simulink model "base_model"  (R2022a)
settings: Solver=ode23t  StartTime=0.0  StopTime=2  RelTol=1e-3
model workspace (MAT data in the model file):
  Kp_MPPT = 1.14714733987
  Ts_Control = 0.0001
  Ts_MPPT = 0.0001
undefined symbols (not defined in the file): Ion, Lithium, load_switch
libraries: spsSeriesRLCBranchLib x13, simulink x6, spsCurrentMeasurementLib x5, spsVoltageMeasurementLib x4, slpidlib x3, spsIGBTDiodeLib x2, spsDiodeLib x2, spsMosfetLib x2, spsPWMGeneratorDCDCLib x2, spsPVArrayLib x2, spsBatteryLib x1, spsIdealSwitchLib x1
settings Model: Creator=drmeg  LastModifiedBy=drmeg
settings SolverCC: ZeroCrossAlgorithm=Adaptive
settings OptimizationCC: ZeroExternalMemoryAtStartup=off  ZeroInternalMemoryAtStartup=off
settings DebuggingCC: MaskedZcDiagnostic=none  IgnoredZcDiagnostic=none  UnconnectedInputMsg=warning  UnconnectedOutputMsg=warning  UnconnectedLineMsg=warning
settings RTWCC: TargetLang=C++  DLArmComputeVersion=19.05
settings GRTTargetCC: TargetLangStandard=C++11 (ISO)  CodeInterfacePackaging=C++ class

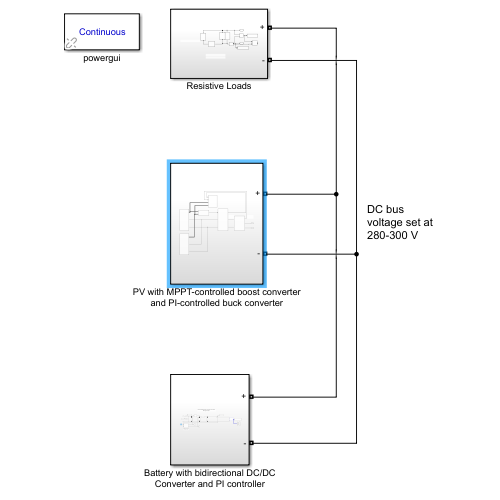
[thumbnail: Simulink's stored preview of the top-level diagram]
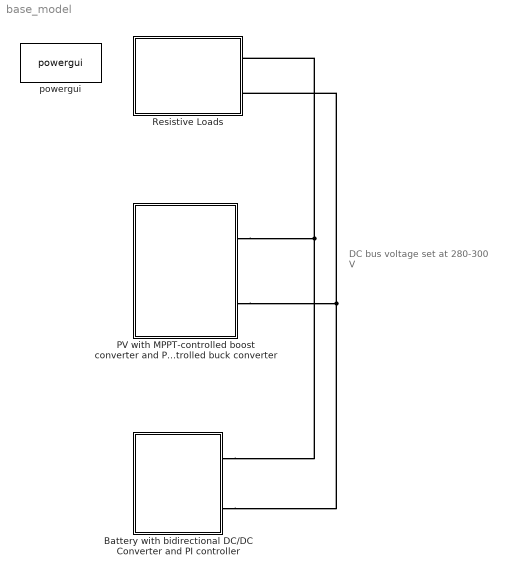
== system base_model ==
  note: DC bus voltage set at
      | 280-300 V
  Battery with bidirectional DC/DC Converter and PI controller : Subsystem
  PV with MPPT-controlled boost converter and PI-controlled buck converter : Subsystem
  Resistive Loads : Subsystem
  powergui : spspowerguiLib/powergui  Priority=1  SimulationMode=Continuous  SampleTime=1e-6  frequency=60  Iterations=50  frequencyindice=0  Pbase=100e6  ErrMax=1e-4  UnitsV=kV  UnitsW=MW  buscounter=0  FunctionMessages=off  echomessages=off  EnableUseOfTLC=off  CurrentSourceSwitches=off  DisableSnubberDevices=off  DisableRonSwitches=off  DisableVfSwitches=off  DisplayEquations=off  AutomaticDiscreteSolvers=off  SolverType=Tustin/Backward Euler (TBE)  Interpol=off  ExternalGateDelay=off  methode=off  Ts=100  x0status=blocks  SPID=on  SwTol=0  HookPort=off  NonlinearTolerance=1e-4  nMaxIteration=100  ContinueOnMaxIteration=off  RestoreLinks=warning  ResistiveCurrentMeasurement=off  Frange=[0:2:500]  Ylog=off  Xlog=on  ShowGrid=off  save=off  variable=ZData  structure=0  ZoomFFT=off  StartTime=0.0  cycles=1  DisplayStyle=1  fundamental=60  FreqAxis=off  MaxFrequency=1000  frequencyindicesteady=1  RmsSteady=1  display=off
  connections:
  Battery with bidirectional DC/DC Converter and PI controller/LConn2 -- Resistive Loads/RConn2 -- PV with MPPT-controlled boost converter and PI-controlled buck converter/RConn2
  Battery with bidirectional DC/DC Converter and PI controller/LConn1 -- Resistive Loads/RConn1 -- PV with MPPT-controlled boost converter and PI-controlled buck converter/RConn1

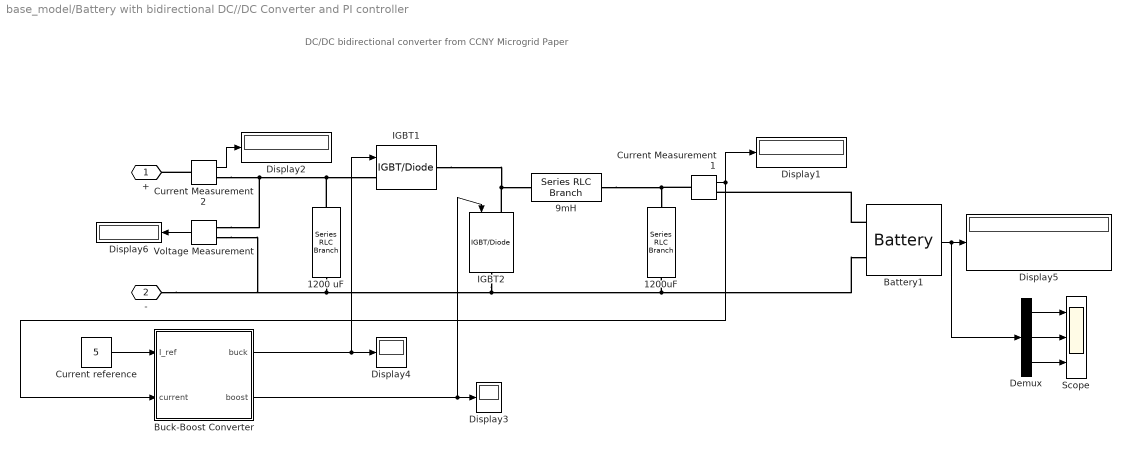
== system base_model/Battery with bidirectional DC//DC Converter and PI controller ==
  note: DC/DC bidirectional converter from CCNY Microgrid Paper
  1200 uF : spsSeriesRLCBranchLib/Series RLC Branch  LConnTagsString=__new0  RConnTagsString=__new0  BranchType=RC  Resistance=0.1  Inductance=3e-3  SetiL0=off  InitialCurrent=0  Capacitance=1200e-6  Setx0=off  InitialVoltage=0  Measurements=None
  1200uF : spsSeriesRLCBranchLib/Series RLC Branch  LConnTagsString=__new0  RConnTagsString=__new0  BranchType=C  Resistance=1  Inductance=3e-3  SetiL0=off  InitialCurrent=0  Capacitance=1200e-6  Setx0=off  InitialVoltage=0  Measurements=None
  9mH : spsSeriesRLCBranchLib/Series RLC Branch  LConnTagsString=__new0  RConnTagsString=__new0  BranchType=L  Resistance=1  Inductance=9e-3  SetiL0=off  InitialCurrent=0  Capacitance=1e-6  Setx0=off  InitialVoltage=0  Measurements=None
  Battery1 : spsBatteryLib/Battery  BatType=Lithium-Ion  ShowTempParam=off  ThermalPreset=no  ShowAgeParam=off  NomV=150  NomQ=80  SOC=100  Batt_Tr=3  PresetModel=on  MaxQ=80  MinV=112.5  FullV=174.5981  Dis_rate=34.7826  R=0.01875  Normal_OP=72.3478  expZone="[162.0579      3.930435]"  current=[1.5 3]  Units=Ampere-hour  Tci=20  NomT=25  T2=0  MaxQ2=2.208  FullV2=3.45  Normal_OP2=2.8  expZone2="[3.22        0.23]"  Rca=0.6  ti=1000  Dp=0  Neq0=0  Tsim=1e6  Ta1=25  Qeol=5.4*0.9  Reol=0.013333*1.2  Char_age=[2.3478, 3]  Dis_age=[2.3478, 10]  N1=1500  N2=10500  N3=1000  N4=1400  Ta2=45  N5=950
  Buck-Boost Converter : Subsystem
  Current Measurement1 : spsCurrentMeasurementLib/Current Measurement  PhasorSimulation=off  OutputType=Complex  PSBequivalent=0
  Current Measurement2 : spsCurrentMeasurementLib/Current Measurement  PhasorSimulation=off  OutputType=Complex  PSBequivalent=0
  Current reference : Constant  Value=5
  Demux : Demux  Outputs=3
  Display{1..6} (6 alike) : Display
      Display5 settings: Format=decimal (Stored Integer)
  IGBT1 : spsIGBTDiodeLib/IGBT//Diode  Ron=1e-3  Rs=1e5  Cs=inf  Measurements=off
  IGBT2 : spsIGBTDiodeLib/IGBT//Diode  Ron=1e-3  Rs=1e5  Cs=inf  Measurements=off
  Scope : Scope  NumInputPorts=3
  Voltage Measurement : spsVoltageMeasurementLib/Voltage Measurement  PhasorSimulation=off  OutputType=Complex  PSBequivalent=0
  + : PMIOPort  Side=Left
  - : PMIOPort  Port=2  Side=Left
  wires:
  Buck-Boost Converter/2(boost) -> Display3/1, IGBT2/1
  Current Measurement1/1 -> Display1/1, Buck-Boost Converter/2(current)
  Buck-Boost Converter/1(buck) -> Display4/1, IGBT1/1
  Current reference/1 -> Buck-Boost Converter/1(I_ref)
  Current Measurement2/1 -> Display2/1
  Battery1/1 -> Demux/1, Display5/1
  Voltage Measurement/1 -> Display6/1
  Demux/3 -> Scope/3
  Demux/2 -> Scope/2
  Demux/1 -> Scope/1
  connections:
  Current Measurement1/LConn1 -- 1200uF/LConn1 -- 9mH/RConn1
  1200uF/RConn1 -- Battery1/LConn2 -- IGBT2/RConn1 -- -/RConn1 -- Voltage Measurement/LConn2 -- 1200 uF/RConn1
  IGBT1/RConn1 -- 9mH/LConn1 -- IGBT2/LConn1
  Current Measurement2/RConn1 -- 1200 uF/LConn1 -- IGBT1/LConn1 -- Voltage Measurement/LConn1
  Battery1/LConn1 -- Current Measurement1/RConn1
  Current Measurement2/LConn1 -- +/RConn1

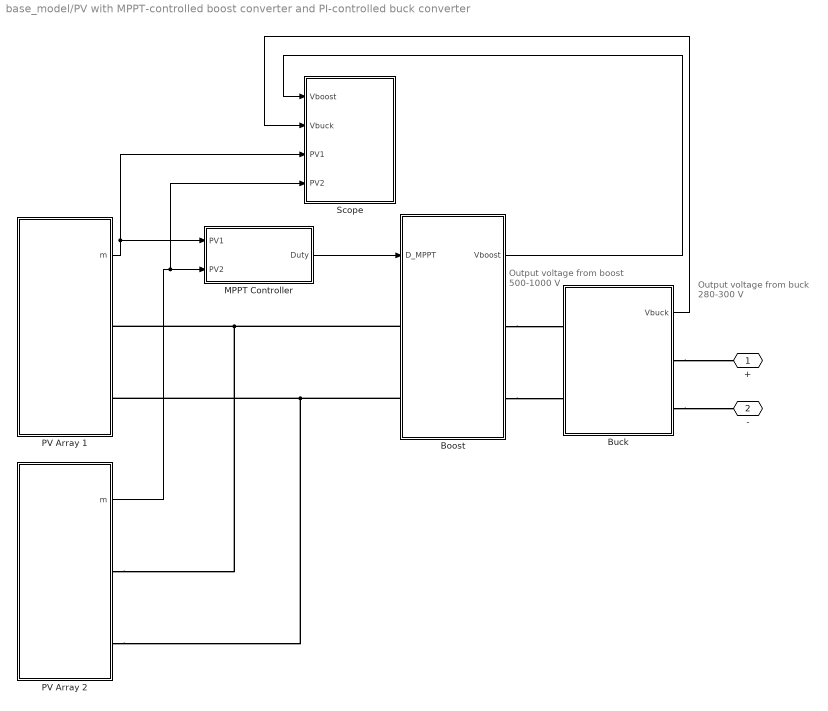
== system base_model/PV with MPPT-controlled boost converter and PI-controlled buck converter ==
  note: Output voltage
      | from boost
      | 500-1000 V
  note: Output voltage
      | from buck
      | 280-300 V
  Boost : Subsystem
  Buck : Subsystem
  MPPT Controller : Subsystem
  PV Array 1 : Subsystem
  PV Array 2 : Subsystem
  Scope : Subsystem
  " +" : PMIOPort  Side=Right
  " -" : PMIOPort  Port=2  Side=Right
  wires:
  PV Array 1/1(m) -> Scope/3(PV1), MPPT Controller/1(PV1)
  MPPT Controller/1(Duty) -> Boost/1(D_MPPT)
  Buck/1(Vbuck) -> Scope/2(Vbuck)
  Boost/1(Vboost) -> Scope/1(Vboost)
  PV Array 2/1(m) -> Scope/4(PV2), MPPT Controller/2(PV2)
  connections:
  Boost/RConn2 -- Buck/LConn2
  Boost/LConn1 -- PV Array 1/RConn1 -- PV Array 2/RConn1
  Boost/LConn2 -- PV Array 2/RConn2 -- PV Array 1/RConn2
  Boost/RConn1 -- Buck/LConn1
  Buck/RConn2 -- " -"/RConn1
  Buck/RConn1 -- " +"/RConn1

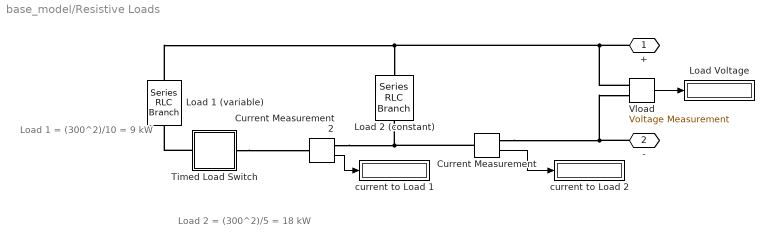
== system base_model/Resistive Loads ==
  note: Load 1 = (300^2)/10 = 9 kW
  note: Load 2 = (300^2)/5 = 18 kW
  Current Measurement : spsCurrentMeasurementLib/Current Measurement  PhasorSimulation=off  OutputType=Complex  PSBequivalent=0
  Current Measurement2 : spsCurrentMeasurementLib/Current Measurement  PhasorSimulation=off  OutputType=Complex  PSBequivalent=0
  Load 1 (variable) : spsSeriesRLCBranchLib/Series RLC Branch  LConnTagsString=__new0  RConnTagsString=__new0  BranchType=RL  Resistance=10  Inductance=1e-3  SetiL0=off  InitialCurrent=0  Capacitance=220e-6  Setx0=off  InitialVoltage=0  Measurements=None
  Load 2 (constant) : spsSeriesRLCBranchLib/Series RLC Branch  LConnTagsString=__new0  RConnTagsString=__new0  BranchType=RL  Resistance=5  Inductance=1e-3  SetiL0=off  InitialCurrent=0  Capacitance=220e-6  Setx0=off  InitialVoltage=0  Measurements=None
  Load Voltage : Display
  Timed Load Switch : Subsystem
  Vload : spsVoltageMeasurementLib/Voltage Measurement  PhasorSimulation=off  OutputType=Complex  PSBequivalent=0
  current to Load 1 : Display
  current to Load 2 : Display
  + : PMIOPort  Side=Right
  - : PMIOPort  Port=2  Side=Right
  wires:
  Vload/1 -> Load Voltage/1
  Current Measurement/1 -> current to Load 2/1
  Current Measurement2/1 -> current to Load 1/1
  connections:
  Vload/LConn1 -- +/RConn1 -- Load 1 (variable)/LConn1 -- Load 2 (constant)/LConn1
  -/RConn1 -- Vload/LConn2 -- Current Measurement/RConn1
  Timed Load Switch/LConn1 -- Load 1 (variable)/RConn1
  Timed Load Switch/RConn1 -- Current Measurement2/LConn1
  Current Measurement/LConn1 -- Load 2 (constant)/RConn1 -- Current Measurement2/RConn1

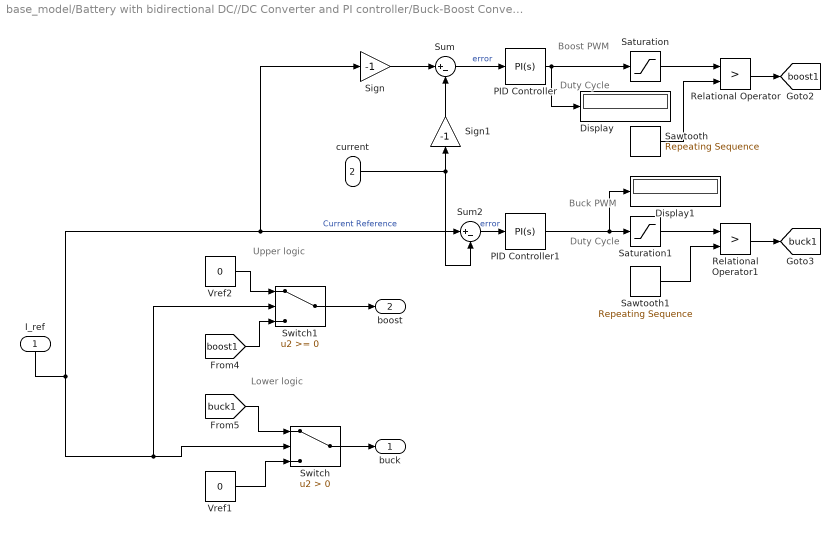
== system base_model/Battery with bidirectional DC//DC Converter and PI controller/Buck-Boost Converter ==
  note: Buck PWM
  note: Duty Cycle
  note: Upper logic
  note: Lower logic
  note: Boost PWM
  note: Duty Cycle
  I_ref : Inport
  current : Inport  Port=2
  Display : Display
  Display1 : Display
  PID Controller : slpidlib/PID Controller  Controller=PI  Form=Parallel  TimeDomain=Continuous-time  UseExternalTs=off  SampleTime=-1  IntegratorMethod=Forward Euler  FilterMethod=Forward Euler  ControllerParametersSource=internal  P=-.1  I=0.02  UseKiTs=off  D=0  N=100  UseFilter=on  TunerSelectOption=Transfer Function Based (PID Tuner App)  InitialConditionSource=internal  InitialConditionForIntegrator=0  InitialConditionForFilter=0  DifferentiatorICPrevScaledInput=0  ExternalReset=none  TrackingMode=off  Kt=1  LimitOutput=off  SatLimitsSource=internal  UpperSaturationLimit=inf  LowerSaturationLimit=-inf  LinearizeAsGain=on  AntiWindupMode=none  Kb=1  POutMin=[]  POutMax=[]  IOutMin=[]  IOutMax=[]  DOutMin=[]  DOutMax=[]  NOutMin=[]  NOutMax=[]  SumOutMin=[]  SumOutMax=[]  SaturationOutMin=[]  SaturationOutMax=[]  PParamMin=[]  PParamMax=[]  IParamMin=[]  IParamMax=[]  DParamMin=[]  DParamMax=[]  NParamMin=[]  NParamMax=[]  KbParamMin=[]  KbParamMax=[]  KtParamMin=[]  KtParamMax=[]  KbOutMin=[]  KbOutMax=[]  KtOutMin=[]  KtOutMax=[]  IntegratorOutMin=[]  IntegratorOutMax=[]  FilterOutMin=[]  FilterOutMax=[]  SumI1OutMin=[]  SumI1OutMax=[]  SumI2OutMin=[]  SumI2OutMax=[]  SumI3OutMin=[]  SumI3OutMax=[]  SumI4OutMin=[]  SumI4OutMax=[]  SumDOutMin=[]  SumDOutMax=[]  DifferentiatorOutMin=[]  DifferentiatorOutMax=[]  FilterDiffOutCoefMin=[]  FilterDiffOutCoefMax=[]  ReciprocalOutMin=[]  ReciprocalOutMax=[]  SumDenOutMin=[]  SumDenOutMax=[]  SumNumOutMin=[]  SumNumOutMax=[]  DivideOutMin=[]  DivideOutMax=[]  UdiffTsProdOutMin=[]  UdiffTsProdOutMax=[]  NTsProdOutMin=[]  NTsProdOutMax=[]  UintegralTsProdOutMin=[]  UintegralTsProdOutMax=[]  UngainTsProdOutMin=[]  UngainTsProdOutMax=[]  IntegratorContinuousStateAttributes=''  IntegratorStateMustResolveToSignalObject=off  IntegratorRTWStateStorageClass=Auto  FilterContinuousStateAttributes=''  FilterStateMustResolveToSignalObject=off  FilterRTWStateStorageClass=Auto  ParallelPVariant=InternalParameters  IdealPVariant=Disabled  IVariant=InternalParameters  DVariant=Disabled  IntegratorVariant=Continuous  SatVariant=Disabled  AWVariant=Passthrough  PCopyVariant=Disabled  TRVariant=Disabled  FdbkBlocksVariant=Forward  IdealPFdbkVariant=Disabled  SatFdbkVariant=Disabled  DerivativeFilterVariant=Disabled  NVariant=Disabled  NCopyVariant=Disabled_SignalSpec  FilterICVariant=Disabled  IntegratorICVariant=InternalICs  ExternalResetVariant=Disabled  TRSumVariant=Passthrough  SumFdbkVariant=Disabled  SumVariant=Sum_PI  TsampFilterVariant=InternalTs  TsampNgainVariant=Passthrough  TsampIntegralVariant=Passthrough  ExternalSaturationOutDataTypeStr=Inherit: Same as second input  aMode=0
  PID Controller1 : slpidlib/PID Controller  Controller=PI  Form=Parallel  TimeDomain=Continuous-time  UseExternalTs=off  SampleTime=-1  IntegratorMethod=Forward Euler  FilterMethod=Forward Euler  ControllerParametersSource=internal  P=0.1  I=0.001  UseKiTs=off  D=0  N=100  UseFilter=on  TunerSelectOption=Transfer Function Based (PID Tuner App)  InitialConditionSource=internal  InitialConditionForIntegrator=0  InitialConditionForFilter=0  DifferentiatorICPrevScaledInput=0  ExternalReset=none  TrackingMode=off  Kt=1  LimitOutput=off  SatLimitsSource=internal  UpperSaturationLimit=inf  LowerSaturationLimit=-inf  LinearizeAsGain=on  AntiWindupMode=none  Kb=1  POutMin=[]  POutMax=[]  IOutMin=[]  IOutMax=[]  DOutMin=[]  DOutMax=[]  NOutMin=[]  NOutMax=[]  SumOutMin=[]  SumOutMax=[]  SaturationOutMin=[]  SaturationOutMax=[]  PParamMin=[]  PParamMax=[]  IParamMin=[]  IParamMax=[]  DParamMin=[]  DParamMax=[]  NParamMin=[]  NParamMax=[]  KbParamMin=[]  KbParamMax=[]  KtParamMin=[]  KtParamMax=[]  KbOutMin=[]  KbOutMax=[]  KtOutMin=[]  KtOutMax=[]  IntegratorOutMin=[]  IntegratorOutMax=[]  FilterOutMin=[]  FilterOutMax=[]  SumI1OutMin=[]  SumI1OutMax=[]  SumI2OutMin=[]  SumI2OutMax=[]  SumI3OutMin=[]  SumI3OutMax=[]  SumI4OutMin=[]  SumI4OutMax=[]  SumDOutMin=[]  SumDOutMax=[]  DifferentiatorOutMin=[]  DifferentiatorOutMax=[]  FilterDiffOutCoefMin=[]  FilterDiffOutCoefMax=[]  ReciprocalOutMin=[]  ReciprocalOutMax=[]  SumDenOutMin=[]  SumDenOutMax=[]  SumNumOutMin=[]  SumNumOutMax=[]  DivideOutMin=[]  DivideOutMax=[]  UdiffTsProdOutMin=[]  UdiffTsProdOutMax=[]  NTsProdOutMin=[]  NTsProdOutMax=[]  UintegralTsProdOutMin=[]  UintegralTsProdOutMax=[]  UngainTsProdOutMin=[]  UngainTsProdOutMax=[]  IntegratorContinuousStateAttributes=''  IntegratorStateMustResolveToSignalObject=off  IntegratorRTWStateStorageClass=Auto  FilterContinuousStateAttributes=''  FilterStateMustResolveToSignalObject=off  FilterRTWStateStorageClass=Auto  ParallelPVariant=InternalParameters  IdealPVariant=Disabled  IVariant=InternalParameters  DVariant=Disabled  IntegratorVariant=Continuous  SatVariant=Disabled  AWVariant=Passthrough  PCopyVariant=Disabled  TRVariant=Disabled  FdbkBlocksVariant=Forward  IdealPFdbkVariant=Disabled  SatFdbkVariant=Disabled  DerivativeFilterVariant=Disabled  NVariant=Disabled  NCopyVariant=Disabled_SignalSpec  FilterICVariant=Disabled  IntegratorICVariant=InternalICs  ExternalResetVariant=Disabled  TRSumVariant=Passthrough  SumFdbkVariant=Disabled  SumVariant=Sum_PI  TsampFilterVariant=InternalTs  TsampNgainVariant=Passthrough  TsampIntegralVariant=Passthrough  ExternalSaturationOutDataTypeStr=Inherit: Same as second input  aMode=0
  Relational Operator : RelationalOperator  Operator=>  OutDataTypeStr=boolean  InputSameDT=off
  Relational Operator1 : RelationalOperator  Operator=>  OutDataTypeStr=boolean  InputSameDT=off
  Saturation : Saturate  UpperLimit=0.9  LowerLimit=0
  Saturation1 : Saturate  UpperLimit=0.9  LowerLimit=0
  Sawtooth : simulink/Sources/Repeating Sequence  rep_seq_t=[0 1/5000]  rep_seq_y=[0 1]
  Sawtooth1 : simulink/Sources/Repeating Sequence  rep_seq_t=[0 1/5000]  rep_seq_y=[0 1]
  Sign : Gain  Gain=-1
  Sign1 : Gain  Gain=-1
  Sum : Sum  Inputs=|+-
  Sum2 : Sum  Inputs=|+-
  Switch : Switch  Criteria=u2 > Threshold  SaturateOnIntegerOverflow=off  InputSameDT=off
  Switch1 : Switch  SaturateOnIntegerOverflow=off  InputSameDT=off
  Vref1 : Constant  Value=0
  Vref2 : Constant  Value=0
  buck : Outport
  boost : Outport  Port=2
  tag scope: boost1=global, buck1=global
  wires:
  Sum/1 -> PID Controller/1  "error"
  Relational Operator/1 -> [boost1]
  Sign/1 -> Sum/1
  PID Controller1/1 -> Display1/1, Saturation1/1
  Sawtooth/1 -> Relational Operator/2
  Sawtooth1/1 -> Relational Operator1/2
  current/1 -> Sum2/2, Sign1/1
  Relational Operator1/1 -> [buck1]
  Sum2/1 -> PID Controller1/1  "error"
  Saturation/1 -> Relational Operator/1
  Saturation1/1 -> Relational Operator1/1
  Vref1/1 -> Switch/3
  Vref2/1 -> Switch1/1
  [boost1] -> Switch1/3
  Switch/1 -> buck/1
  [buck1] -> Switch/1
  I_ref/1 -> Switch1/2, Switch/2, Sign/1, Sum2/1  "Current Reference"
  Sign1/1 -> Sum/2
  PID Controller/1 -> Display/1, Saturation/1
  Switch1/1 -> boost/1

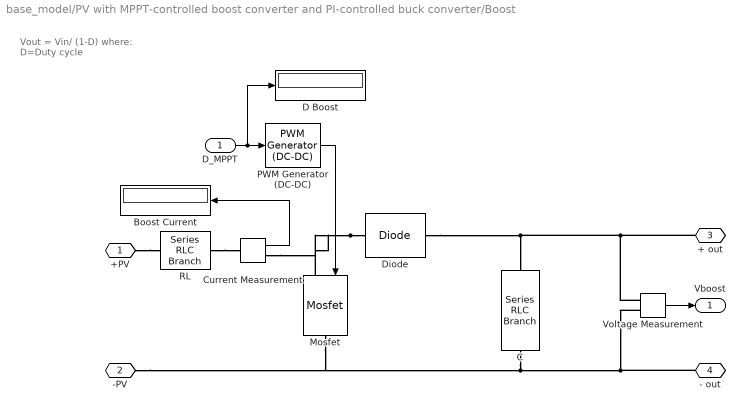
== system base_model/PV with MPPT-controlled boost converter and PI-controlled buck converter/Boost ==
  note: Vout = Vin/ (1-D)
      | where: D=Duty cycle
  D_MPPT : Inport
  Boost Current : Display
  C : spsSeriesRLCBranchLib/Series RLC Branch  LConnTagsString=__new0  RConnTagsString=__new0  BranchType=RC  Resistance=1e-3  Inductance=1e-3  SetiL0=off  InitialCurrent=0  Capacitance=4.394e-4  Setx0=off  InitialVoltage=0  Measurements=None
  Current Measurement : spsCurrentMeasurementLib/Current Measurement  PhasorSimulation=off  OutputType=Complex  PSBequivalent=0
  D Boost : Display
  Diode : spsDiodeLib/Diode  Ron=1e-3  Lon=0  Vf=0.8  IC=0  UseSnubber=0  Rs=500  Cs=250e-9  Measurements=off
  Mosfet : spsMosfetLib/Mosfet  Ron=1e-3  Lon=0  Rd=1e-3  Vfd=0  IC=0  Rs=inf  Cs=inf  Measurements=off
  PWM Generator (DC-DC) : spsPWMGeneratorDCDCLib/PWM Generator (DC-DC)  Fsw=5000  Ts=0
  RL : spsSeriesRLCBranchLib/Series RLC Branch  LConnTagsString=__new0  RConnTagsString=__new0  BranchType=RL  Resistance=1e-3  Inductance=2.269e-3  SetiL0=off  InitialCurrent=0  Capacitance=1e-6  Setx0=off  InitialVoltage=0  Measurements=None
  Voltage Measurement : spsVoltageMeasurementLib/Voltage Measurement  PhasorSimulation=off  OutputType=Complex  PSBequivalent=0
  +PV : PMIOPort  Side=Left
  -PV : PMIOPort  Port=2  Side=Left
  " + out" : PMIOPort  Port=3  Side=Right
  " - out" : PMIOPort  Port=4  Side=Right
  Vboost : Outport
  wires:
  Voltage Measurement/1 -> Vboost/1
  Current Measurement/1 -> Boost Current/1
  PWM Generator (DC-DC)/1 -> Mosfet/1
  D_MPPT/1 -> D Boost/1, PWM Generator (DC-DC)/1
  connections:
  Voltage Measurement/LConn2 -- " - out"/RConn1 -- Mosfet/RConn1 -- -PV/RConn1 -- C/RConn1
  Voltage Measurement/LConn1 -- " + out"/RConn1 -- C/LConn1 -- Diode/RConn1
  Diode/LConn1 -- Mosfet/LConn1 -- Current Measurement/RConn1
  +PV/RConn1 -- RL/LConn1
  RL/RConn1 -- Current Measurement/LConn1

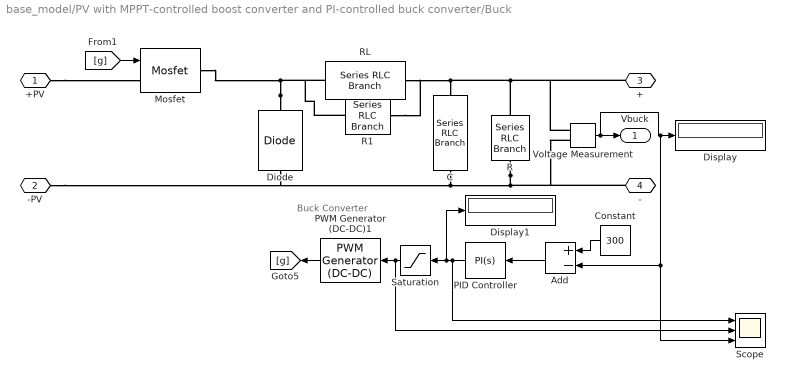
== system base_model/PV with MPPT-controlled boost converter and PI-controlled buck converter/Buck ==
  note: Buck Converter
  Add : Sum  Inputs=+-
  C : spsSeriesRLCBranchLib/Series RLC Branch  LConnTagsString=__new0  RConnTagsString=__new0  BranchType=RC  Resistance=1e-3  Inductance=1e-3  SetiL0=off  InitialCurrent=0  Capacitance=1.25e-4  Setx0=off  InitialVoltage=0  Measurements=None
  Constant : Constant  Value=300
  Diode : spsDiodeLib/Diode  Ron=1e-3  Lon=0  Vf=0  IC=0  UseSnubber=0  Rs=inf  Cs=inf  Measurements=off
  Display : Display
  Display1 : Display
  Mosfet : spsMosfetLib/Mosfet  Ron=1e-3  Lon=0  Rd=1e-3  Vfd=0  IC=0  Rs=inf  Cs=inf  Measurements=off
  PID Controller : slpidlib/PID Controller  Controller=PI  Form=Parallel  TimeDomain=Continuous-time  UseExternalTs=off  SampleTime=-1  IntegratorMethod=Forward Euler  FilterMethod=Forward Euler  ControllerParametersSource=internal  P=0.03  I=0.001  UseKiTs=off  D=0  N=100  UseFilter=on  TunerSelectOption=Transfer Function Based (PID Tuner App)  InitialConditionSource=internal  InitialConditionForIntegrator=0  InitialConditionForFilter=0  DifferentiatorICPrevScaledInput=0  ExternalReset=none  TrackingMode=off  Kt=1  LimitOutput=off  SatLimitsSource=internal  UpperSaturationLimit=inf  LowerSaturationLimit=-inf  LinearizeAsGain=on  AntiWindupMode=none  Kb=1  POutMin=[]  POutMax=[]  IOutMin=[]  IOutMax=[]  DOutMin=[]  DOutMax=[]  NOutMin=[]  NOutMax=[]  SumOutMin=[]  SumOutMax=[]  SaturationOutMin=[]  SaturationOutMax=[]  PParamMin=[]  PParamMax=[]  IParamMin=[]  IParamMax=[]  DParamMin=[]  DParamMax=[]  NParamMin=[]  NParamMax=[]  KbParamMin=[]  KbParamMax=[]  KtParamMin=[]  KtParamMax=[]  KbOutMin=[]  KbOutMax=[]  KtOutMin=[]  KtOutMax=[]  IntegratorOutMin=[]  IntegratorOutMax=[]  FilterOutMin=[]  FilterOutMax=[]  SumI1OutMin=[]  SumI1OutMax=[]  SumI2OutMin=[]  SumI2OutMax=[]  SumI3OutMin=[]  SumI3OutMax=[]  SumI4OutMin=[]  SumI4OutMax=[]  SumDOutMin=[]  SumDOutMax=[]  DifferentiatorOutMin=[]  DifferentiatorOutMax=[]  FilterDiffOutCoefMin=[]  FilterDiffOutCoefMax=[]  ReciprocalOutMin=[]  ReciprocalOutMax=[]  SumDenOutMin=[]  SumDenOutMax=[]  SumNumOutMin=[]  SumNumOutMax=[]  DivideOutMin=[]  DivideOutMax=[]  UdiffTsProdOutMin=[]  UdiffTsProdOutMax=[]  NTsProdOutMin=[]  NTsProdOutMax=[]  UintegralTsProdOutMin=[]  UintegralTsProdOutMax=[]  UngainTsProdOutMin=[]  UngainTsProdOutMax=[]  IntegratorContinuousStateAttributes=''  IntegratorStateMustResolveToSignalObject=off  IntegratorRTWStateStorageClass=Auto  FilterContinuousStateAttributes=''  FilterStateMustResolveToSignalObject=off  FilterRTWStateStorageClass=Auto  ParallelPVariant=InternalParameters  IdealPVariant=Disabled  IVariant=InternalParameters  DVariant=Disabled  IntegratorVariant=Continuous  SatVariant=Disabled  AWVariant=Passthrough  PCopyVariant=Disabled  TRVariant=Disabled  FdbkBlocksVariant=Forward  IdealPFdbkVariant=Disabled  SatFdbkVariant=Disabled  DerivativeFilterVariant=Disabled  NVariant=Disabled  NCopyVariant=Disabled_SignalSpec  FilterICVariant=Disabled  IntegratorICVariant=InternalICs  ExternalResetVariant=Disabled  TRSumVariant=Passthrough  SumFdbkVariant=Disabled  SumVariant=Sum_PI  TsampFilterVariant=InternalTs  TsampNgainVariant=Passthrough  TsampIntegralVariant=Passthrough  ExternalSaturationOutDataTypeStr=Inherit: Same as second input  aMode=0
  PWM Generator (DC-DC)1 : spsPWMGeneratorDCDCLib/PWM Generator (DC-DC)  Fsw=1000  Ts=0
  R : spsSeriesRLCBranchLib/Series RLC Branch  LConnTagsString=__new0  RConnTagsString=__new0  BranchType=R  Resistance=10  Inductance=1e-3  SetiL0=off  InitialCurrent=0  Capacitance=220e-6  Setx0=off  InitialVoltage=0  Measurements=None
  R1 : spsSeriesRLCBranchLib/Series RLC Branch  LConnTagsString=__new0  RConnTagsString=__new0  BranchType=R  Resistance=1e6  Inductance=1e-3  SetiL0=off  InitialCurrent=0  Capacitance=220e-6  Setx0=off  InitialVoltage=0  Measurements=None
  RL : spsSeriesRLCBranchLib/Series RLC Branch  LConnTagsString=__new0  RConnTagsString=__new0  BranchType=RL  Resistance=1e-3  Inductance=20e-3  SetiL0=off  InitialCurrent=5  Capacitance=1e-6  Setx0=off  InitialVoltage=0  Measurements=None
  Saturation : Saturate  UpperLimit=1  LowerLimit=0
  Scope : Scope  NumInputPorts=3
  Voltage Measurement : spsVoltageMeasurementLib/Voltage Measurement  PhasorSimulation=off  OutputType=Complex  PSBequivalent=0
  +PV : PMIOPort  Side=Left
  -PV : PMIOPort  Port=2  Side=Left
  " +" : PMIOPort  Port=3  Side=Right
  " -" : PMIOPort  Port=4  Side=Right
  Vbuck : Outport
  wires:
  Add/1 -> PID Controller/1
  PWM Generator (DC-DC)1/1 -> [g]
  [g] -> Mosfet/1
  Voltage Measurement/1 -> Vbuck/1, Scope/3, Add/2, Display/1
  PID Controller/1 -> Scope/1, Saturation/1, Display1/1
  Saturation/1 -> Scope/2, PWM Generator (DC-DC)1/1
  Constant/1 -> Add/1
  connections:
  Diode/RConn1 -- R1/RConn1 -- RL/LConn1 -- Mosfet/RConn1
  R/RConn1 -- -PV/RConn1 -- Diode/LConn1 -- C/RConn1 -- " -"/RConn1 -- Voltage Measurement/LConn2
  C/LConn1 -- R1/LConn1 -- RL/RConn1 -- R/LConn1 -- " +"/RConn1 -- Voltage Measurement/LConn1
  +PV/RConn1 -- Mosfet/LConn1

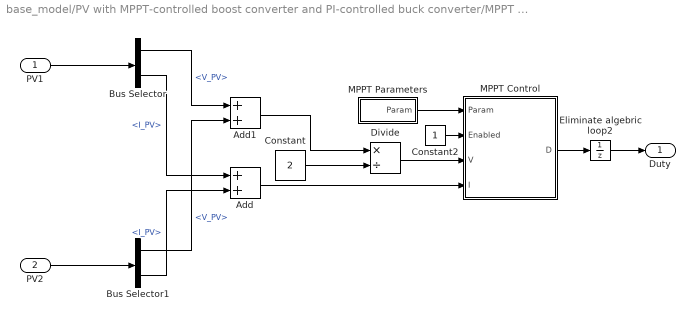
== system base_model/PV with MPPT-controlled boost converter and PI-controlled buck converter/MPPT Controller ==
  PV1 : Inport
  PV2 : Inport  Port=2
  Add : Sum
  Add1 : Sum
  Bus Selector : BusSelector  OutputSignals=V_PV,I_PV
  Bus Selector1 : BusSelector  OutputSignals=V_PV,I_PV
  Constant : Constant  Value=2
  Constant2 : Constant
  Divide : Product  Inputs=*/
  Eliminate algebric loop2 : UnitDelay  InitialCondition=0.485  SampleTime=Ts_Control  HasFrameUpgradeWarning=on
  MPPT Parameters : Subsystem
  "MPPT Control  " : MATLAB Function  TreatAsAtomicUnit=on
  Duty : Outport
  wires:
  Bus Selector/1 -> Add1/1  "<V_PV>"
  Bus Selector1/2 -> Add/2  "<I_PV>"
  Constant/1 -> Divide/2
  Bus Selector1/1 -> Add1/2  "<V_PV>"
  Bus Selector/2 -> Add/1  "<I_PV>"
  Add/1 -> "MPPT Control  "/4(I)
  Constant2/1 -> "MPPT Control  "/2(Enabled)
  Eliminate algebric loop2/1 -> Duty/1
  MPPT Parameters/1(Param) -> "MPPT Control  "/1(Param)
  Add1/1 -> Divide/1
  "MPPT Control  "/1(D) -> Eliminate algebric loop2/1
  PV2/1 -> Bus Selector1/1
  PV1/1 -> Bus Selector/1
  Divide/1 -> "MPPT Control  "/3(V)

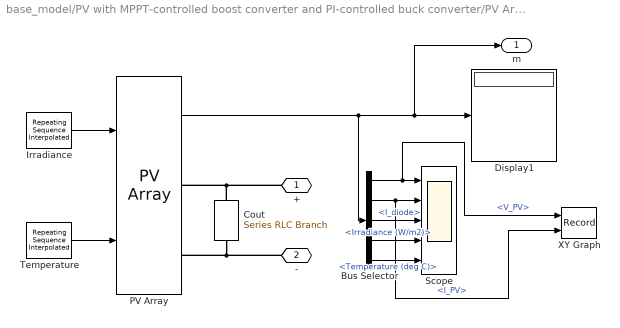
== system base_model/PV with MPPT-controlled boost converter and PI-controlled buck converter/PV Array 1 ==
  Bus Selector : BusSelector  OutputSignals=V_PV,I_PV,I_diode,Irradiance (W/m2),Temperature (deg C)
  Cout : spsSeriesRLCBranchLib/Series RLC Branch  LConnTagsString=__new0  RConnTagsString=__new0  BranchType=RC  Resistance=1e-4  Inductance=2e-3  SetiL0=off  InitialCurrent=0  Capacitance=200e-7  Setx0=off  InitialVoltage=0  Measurements=None
  Display1 : Display
  Irradiance : simulink/Sources/Repeating Sequence Interpolated  OutValues=Irradiance  TimeValues=Time  LookUpMeth=Interpolation-Use End Values  tsamp=0.01  OutMin=[]  OutMax=[]  OutDataTypeStr=double  OutputDataTypeScalingMode=double  OutDataType=fixdt(0,8)  OutScaling=2^-10
  PV Array : spsPVArrayLib/PV Array  Npar=10  Nser=10  PlotType=array @ 1000 W/m2 & specified temperatures  S_vec="[ 1000  500  100 ]"  Temp_C_vec="[ 45 25  ]"  ModuleName=Canadian Solar Inc. CS6P-250P  PlotWhenSelected=off  Pm=249.83  Ncell=60  Voc=37.2  Isc=8.87  Vm=30.1  Im=8.3  beta_Voc_pc=-0.301  alpha_Isc_pc=0.038997  beta_Voc=-0.11197  alpha_Isc=0.003459  IL=8.8849  I0=3.0928e-11  nI=0.91537  Rsh=202.8148  Rs=0.34115  RobustModel=off  RobustCellTemperature=313.3991  BAL=on  Tc=1e-6  Tfilter=5e-5
  Scope : Scope  NumInputPorts=5
  Temperature : simulink/Sources/Repeating Sequence Interpolated  OutValues=Temp  TimeValues=Time  LookUpMeth=Interpolation-Use End Values  tsamp=0.01  OutMin=[]  OutMax=[]  OutDataTypeStr=double  OutputDataTypeScalingMode=double  OutDataType=fixdt(0,8)  OutScaling=2^-10
  XY Graph : Record  FileSettingsInternal="{\"entries\":[{\"content\":{\"excelSettings\":{\"content\":{},\"type\":\"Streamout.ExcelSettings\"}},\"type\":\"Streamout.FileSettingStorage\",\"uuid\":\"d9476bb8-9f6a-4bbf-8cee-e025e801ffd4\"}],\"packageUris\":[\"http://schema.mathworks.com/mf0/streamout_blocks/R2020a\"],\"version\":\"1.0\"}"  Layout=[1 1]  SignalsInternal="{\"entries\":[{\"content\":{\"signals\":[{\"content\":{\"blockPath\":[\"base_model/PV with MPPT-controlled boost converter and PI-controlled buck converter/PV Array 1/XY Graph\"],\"channel\":[],\"dimensions\":[1],\"domain\":\"base_model/PV with MPPT-controlled boost converter and PI-controlled buck converter/PV Array 1/XY Graph\",\"lineColor\":\"#0072bd\",\"plots\":[],\"port\":1,\"sid\":[\"\"],\"signalID\":22100,\"signalName\":\"<V_PV>\"},\"type\":\"RecordBlkView.Signal\",\"uuid\":\"75866728-844d-446b-9991-5566aed4532f\"},{\"content\":{\"blockPath\":[\"base_model/PV with MPPT-controlled boost converter and PI-controlled buck converter/PV Array 1/XY Graph\"],\"channel\":[],\"dimensions\":[1],\"domain\":\"base_model/PV with MPPT-controlled boost converter and PI-controlled buck converter/PV Array 1/XY Graph\",\"lineColor\":\"#d95319\",\"plots\":[],\"port\":2,\"sid\":[\"\"],\"signalID\":22104,\"signalName\":\"<I_PV>\"},\"type\":\"RecordBlkView.Signal\",\"uuid\":\"04a55489-6471-4aa9-a56e-5bbd09e5c0be\"}]},\"type\":\"RecordBlkView.InputSignals\",\"uuid\":\"0630b466-16d7-466f-8953-e1623988410c\"}],\"packageUris\":[\"http://schema.mathworks.com/mf0/streamout_blocks/R2020a\"],\"version\":\"1.0\"}"  VisualizationBindings="{\"xyplotplugin\":{\"info\":[{\"series\":[],\"subplotID\":1}]}}"  CompatibilityTag=XY
  + : PMIOPort  Side=Right
  - : PMIOPort  Port=2  Side=Right
  m : Outport
  wires:
  Irradiance/1 -> PV Array/1
  Temperature/1 -> PV Array/2
  Bus Selector/3 -> Scope/3  "<I_diode>"
  PV Array/1 -> Bus Selector/1, m/1, Display1/1
  Bus Selector/4 -> Scope/4  "<Irradiance (W/m2)>"
  Bus Selector/2 -> XY Graph/2, Scope/2  "<I_PV>"
  Bus Selector/5 -> Scope/5  "<Temperature (deg C)>"
  Bus Selector/1 -> XY Graph/1, Scope/1  "<V_PV>"
  connections:
  +/RConn1 -- Cout/LConn1 -- PV Array/RConn1
  -/RConn1 -- Cout/RConn1 -- PV Array/RConn2

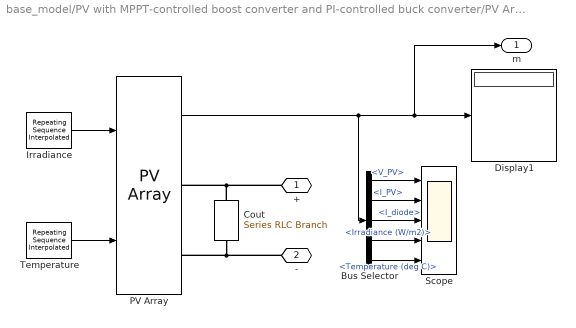
== system base_model/PV with MPPT-controlled boost converter and PI-controlled buck converter/PV Array 2 ==
  Bus Selector : BusSelector  OutputSignals=V_PV,I_PV,I_diode,Irradiance (W/m2),Temperature (deg C)
  Cout : spsSeriesRLCBranchLib/Series RLC Branch  LConnTagsString=__new0  RConnTagsString=__new0  BranchType=RC  Resistance=1e-4  Inductance=2e-3  SetiL0=off  InitialCurrent=0  Capacitance=200e-7  Setx0=off  InitialVoltage=0  Measurements=None
  Display1 : Display
  Irradiance : simulink/Sources/Repeating Sequence Interpolated  OutValues=Irradiance  TimeValues=Time  LookUpMeth=Interpolation-Use End Values  tsamp=0.01  OutMin=[]  OutMax=[]  OutDataTypeStr=double  OutputDataTypeScalingMode=double  OutDataType=fixdt(0,8)  OutScaling=2^-10
  PV Array : spsPVArrayLib/PV Array  Npar=10  Nser=10  PlotType=array @ 1000 W/m2 & specified temperatures  S_vec="[ 1000  500  100 ]"  Temp_C_vec="[ 45 25  ]"  ModuleName=Canadian Solar Inc. CS6P-250P  PlotWhenSelected=off  Pm=249.83  Ncell=60  Voc=37.2  Isc=8.87  Vm=30.1  Im=8.3  beta_Voc_pc=-0.301  alpha_Isc_pc=0.038997  beta_Voc=-0.11197  alpha_Isc=0.003459  IL=8.8849  I0=3.0928e-11  nI=0.91537  Rsh=202.8148  Rs=0.34115  RobustModel=off  RobustCellTemperature=313.3991  BAL=on  Tc=1e-6  Tfilter=5e-5
  Scope : Scope  NumInputPorts=5
  Temperature : simulink/Sources/Repeating Sequence Interpolated  OutValues=Temp  TimeValues=Time  LookUpMeth=Interpolation-Use End Values  tsamp=0.01  OutMin=[]  OutMax=[]  OutDataTypeStr=double  OutputDataTypeScalingMode=double  OutDataType=fixdt(0,8)  OutScaling=2^-10
  + : PMIOPort  Side=Right
  - : PMIOPort  Port=2  Side=Right
  m : Outport
  wires:
  Irradiance/1 -> PV Array/1
  Temperature/1 -> PV Array/2
  Bus Selector/3 -> Scope/3  "<I_diode>"
  PV Array/1 -> Bus Selector/1, m/1, Display1/1
  Bus Selector/4 -> Scope/4  "<Irradiance (W/m2)>"
  Bus Selector/2 -> Scope/2  "<I_PV>"
  Bus Selector/5 -> Scope/5  "<Temperature (deg C)>"
  Bus Selector/1 -> Scope/1  "<V_PV>"
  connections:
  +/RConn1 -- Cout/LConn1 -- PV Array/RConn1
  -/RConn1 -- Cout/RConn1 -- PV Array/RConn2

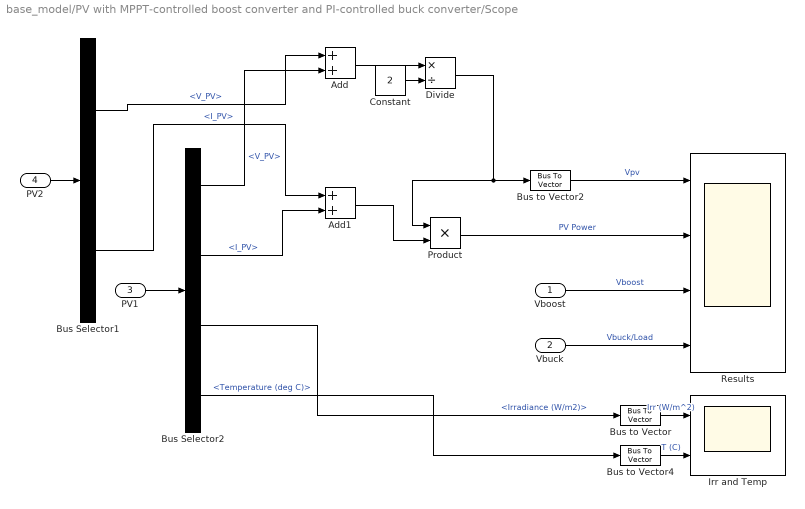
== system base_model/PV with MPPT-controlled boost converter and PI-controlled buck converter/Scope ==
  Vboost : Inport
  Vbuck : Inport  Port=2
  PV1 : Inport  Port=3
  PV2 : Inport  Port=4
  Add : Sum
  Add1 : Sum
  Bus Selector1 : BusSelector  OutputSignals=V_PV,I_PV
  Bus Selector2 : BusSelector  OutputSignals=V_PV,I_PV,Irradiance (W/m2),Temperature (deg C)
  Bus to Vector : BusToVector
  Bus to Vector2 : BusToVector
  Bus to Vector4 : BusToVector
  Constant : Constant  Value=2
  Divide : Product  Inputs=*/
  Irr and Temp : Scope  NumInputPorts=2
  Product : Product
  Results : Scope  NumInputPorts=4
  wires:
  Add/1 -> Divide/1
  Divide/1 -> Bus to Vector2/1, Product/1
  Bus Selector2/2 -> Add1/2  "<I_PV>"
  Constant/1 -> Divide/2
  Add1/1 -> Product/2
  Bus Selector1/1 -> Add/1  "<V_PV>"
  PV2/1 -> Bus Selector1/1
  Bus Selector2/3 -> Bus to Vector/1  "<Irradiance (W/m2)>"
  Bus Selector2/4 -> Bus to Vector4/1  "<Temperature (deg C)>"
  Vboost/1 -> Results/3  "Vboost"
  Bus to Vector4/1 -> Irr and Temp/2  "T (C)"
  Vbuck/1 -> Results/4  "Vbuck/Load"
  Bus to Vector2/1 -> Results/1  "Vpv"
  PV1/1 -> Bus Selector2/1
  Bus to Vector/1 -> Irr and Temp/1  "Irr (W/m^2)"
  Bus Selector1/2 -> Add1/1  "<I_PV>"
  Bus Selector2/1 -> Add/2  "<V_PV>"
  Product/1 -> Results/2  "PV Power"

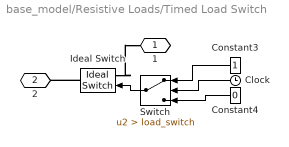
== system base_model/Resistive Loads/Timed Load Switch ==
  Clock : Clock
  Constant3 : Constant
  Constant4 : Constant  Value=0
  Ideal Switch : spsIdealSwitchLib/Ideal Switch  Ron=0.001  Lon=0  IC=0  Rs=1e5  Cs=inf  Measurements=off
  Switch : Switch  Criteria=u2 > Threshold  Threshold=load_switch  SaturateOnIntegerOverflow=off  InputSameDT=off
  1 : PMIOPort  Side=Left
  2 : PMIOPort  Port=2  Side=Right
  wires:
  Constant4/1 -> Switch/3
  Constant3/1 -> Switch/1
  Switch/1 -> Ideal Switch/1
  Clock/1 -> Switch/2
  connections:
  Ideal Switch/LConn1 -- 1/RConn1
  Ideal Switch/RConn1 -- 2/RConn1

== system base_model/PV with MPPT-controlled boost converter and PI-controlled buck converter/MPPT Controller/MPPT Parameters ==
  note: Upper limit for D (Dmax)
  note: Increment value used to increase/decrease (DeltaD)
  note: Initial value for D output (Dinit)
  note: (D = Boost converter duty cycle)
  note: Lower limit for D (Dmax)
  note: Parameters for Perturb and Observe Algorithm:
  Iph_ : Constant  Value=0.495
  Iph_1 : Constant
  Iph_2 : Constant  Value=0
  Iph_3 : Constant  Value=1e-9
  Mux : Mux
  Param : Outport  VectorParamsAs1DForOutWhenUnconnected=off
  wires:
  Iph_/1 -> Mux/1
  Iph_1/1 -> Mux/2
  Iph_2/1 -> Mux/3
  Iph_3/1 -> Mux/4
  Mux/1 -> Param/1

== matlab function base_model/PV with MPPT-controlled boost converter and PI-controlled buck converter/MPPT Controller/MPPT Control   ==
  settings: updateMethod=DISCRETE  sampleTime=Ts_Control
  data: Param input; Enabled input; V input =V; I input; D output
% Function name is called PandO because the MPPT controller duty cycle D is
% determined with a perturb and observe algorithm.

function D  = PandO(Param, Enabled, V, I)

%%% OUTPUTS %%%
% D output = Duty cycle of the boost converter (value between 0 and 1)

%%% INPUTS %%%
% Enabled input = 1 to enable the MPPT controller (assuming always enabled)
% V input = PV array terminal voltage (V)
% I input = PV array current (A)
% Parameter Inputs:
Dinit = Param(1);  % Initial value for D output
Dmax = Param(2);   % Maximum value for D
Dmin = Param(3);   % Minimum value for D
deltaD = Param(4); % Increment value used to increase/decrease the duty cycle D
% ( increasing D = decreasing Vref )
%

%%% PERSISTENT VARIABLES %%%
% These are local variables that you can pass back into a function
persistent Vold Pold Dold;

%%% FUNCTION EQUATIONS %%%

% Set initial value of persistent variables at zero
if isempty(Vold)
    Vold = 0;
    Pold = 0;
    Dold = Dinit;
end

% Define power P = Voltage * Current
P = V*I;

% Define changes in Volage and Power as current value - previous value
dV = V - Vold;
dP = P - Pold;

% This logic says the duty cycle is changed only for non-zero changes in
% power and if the MPPT controller is enabled. If the change in power and
% voltage are both negative, then duty cycle D decreases by user-determined
% increment. If power decreased but voltage increased, then D increases.
% If power increased but voltage decreased, D increases and if power increased
% and volage increased then D decreases. Basically if the change in power and
% voltage are the same sign, D goes down. Different sign and D goes up. The
% goal in any case is to increase P or keep P at the maximum if it is already.

if dP ~= 0 && Enabled ~=0
    if dP < 0
        if dV < 0
            D = Dold - deltaD;
        else
            D = Dold + deltaD;
        end
    else
        if dV < 0
            D = Dold + deltaD;
        else
            D = Dold - deltaD;
        end
    end
else D=Dold;
end

% If the new D is outside of its constraints, then return to previous value
if D >= Dmax || D<= Dmin
    D=Dold;
end

% Assign new duty cycle, voltage, and power as 'old' values for next timestep
Dold=D;
Vold=V;
Pold=P;
